simulink model "vendingmachine"  (R2018b)
settings: Solver=VariableStepAuto  StartTime=0.0  StopTime=10.0  RelTol=1e-3
libraries: simulink x1
settings Model: Creator=ilab  LastModifiedBy=ilab

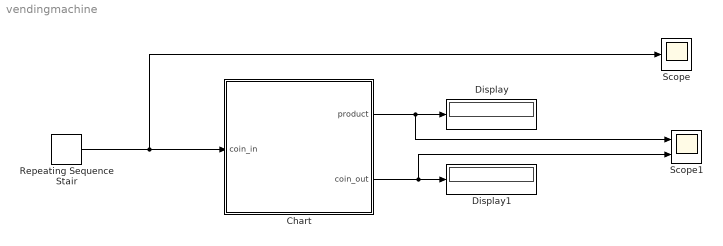
== system vendingmachine ==
  Chart : Stateflow chart  TreatAsAtomicUnit=on  SystemSampleTime=1
  Display : Display
  Display1 : Display
  Repeating Sequence Stair : simulink/Sources/Repeating Sequence Stair  OutValues=[0 50 100 100 100 50]  tsamp=1  OutMin=[]  OutMax=[]  OutDataTypeStr=double  OutputDataTypeScalingMode=double  OutDataType=fixdt(0,8)  ConRadixGroup=Best Precision: Vector-wise  OutScaling=2^-12
  Scope : Scope
  Scope1 : Scope  NumInputPorts=2
  wires:
  Repeating Sequence Stair/1 -> Scope/1, Chart/1(coin_in)
  Chart/1(product) -> Scope1/1, Display/1
  Chart/2(coin_out) -> Scope1/2, Display1/1

== stateflow chart vendingmachine/Chart ==
  state en0
  state en100
  state en50
  (default) -> en0 : {product=0;coin_out=0;}
  en0 -> en0 [order 3] : {product=0;coin_out=0;}
  en100 -> en0 [order 2] : [coin_in==100]{product=1;coin_out=1;}
  en0 -> en50 [order 1] : [coin_in==50]{product=0;coin_out=0;}
  en100 -> en0 [order 1] : [coin_in==50]{product=1;coin_out=0;}
  en50 -> en0 [order 1] : [coin_in==100]{product=1;coin_out=0;}
  en0 -> en100 [order 2] : [coin_in==100]{product=0;coin_out=0;}
  en50 -> en50 [order 3] : {product=0;coin_out=0;}
  en100 -> en100 [order 3] : {product=0;coin_out=0;}
  en50 -> en100 [order 2] : [coin_in==50]{product=0;coin_out=0;}
  data: product output; coin_in input; coin_out output
